simulink model "motor_foc"  (R2023b)
settings: Solver=FixedStepDiscrete  StartTime=0.0  StopTime=4  FixedStep=Ts  RelTol=1e-3  EnableMultiTasking=on
PreLoadFcn:
  | addpath(pwd);
InitFcn:
  | mc_init;
values from neighbouring files (symbols this model uses):
  ADC_Trigger = ADC_Trigger_Top    (= 1)    [mc_init.m]
  B = 0.000    (= 0)    [mc_init.m]
  Cdc = 470e-9    (= 4.7e-07)    [mc_init.m]
  Cphase = 2.2e-9    (= 2.2e-09)    [mc_init.m]
  enc_cpr = 4095    [mc_init.m]
  J = 0.020    (= 0.02)    [mc_init.m]
  Ld = 0.043e-3    (= 4.3e-05)    [mc_init.m]
  Lq = 0.060e-3    (= 6e-05)    [mc_init.m]
  n_polePairs = 5    [mc_init.m]
  PWM_Half_Cnt = PWM_Cnt/2    (= 3000)    [mc_init.m]
  R1 = 400e3    (= 400000)    [mc_init.m]
  R2 = 12e3    (= 12000)    [mc_init.m]
  Rdc = 2000    [mc_init.m]
  Rphase = 120    [mc_init.m]
  Rs = 0.015    [mc_init.m]
  Rshut = 0.001    [mc_init.m]
  TIMER_PWM_MODE = PWM_MODE1    (= 1)    [mc_init.m]
  Ts = 5e-7    (= 5e-07)    [mc_init.m]
  Ts_ctrl = 100e-6    (= 0.0001)    [mc_init.m]
  Udc = 96    [mc_init.m]
  Vbus_C = 3000e-6    (= 0.003)    [mc_init.m]
undefined symbols (not defined in the file or in its folder): Phase_Vol_R1
libraries: spsSeriesRLCBranchLib x9, spsIGBTDiodeLib x6, spsParallelRLCBranchLib x4, spsVoltageMeasurementLib x4, simulink x3, spsControlledVoltageSourceLib x1, spsPermanentMagnetSynchronousMachineLib x1, sps_lib x1
settings Model: Creator=kevin  LastModifiedBy=huhui
settings SolverCC: AlgebraicLoopSolver=TrustRegion  AutoInsertRateTranBlk=on
settings DebuggingCC: UnconnectedInputMsg=warning  UnconnectedOutputMsg=warning  UnconnectedLineMsg=warning
settings ModelReferenceCC: EnableRefExpFcnMdlSchedulingChecks=on
settings RTWCC: DLArmComputeVersion=19.05

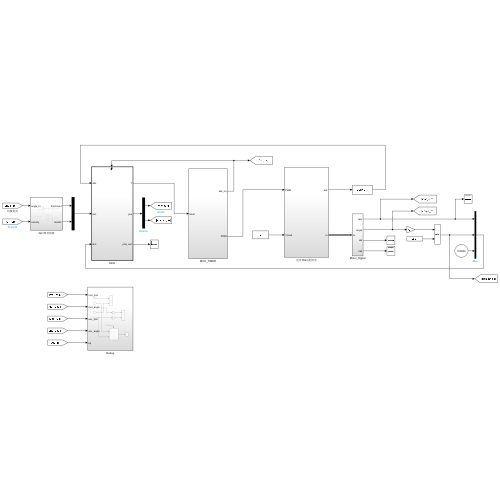
[thumbnail: Simulink's stored preview of the top-level diagram]
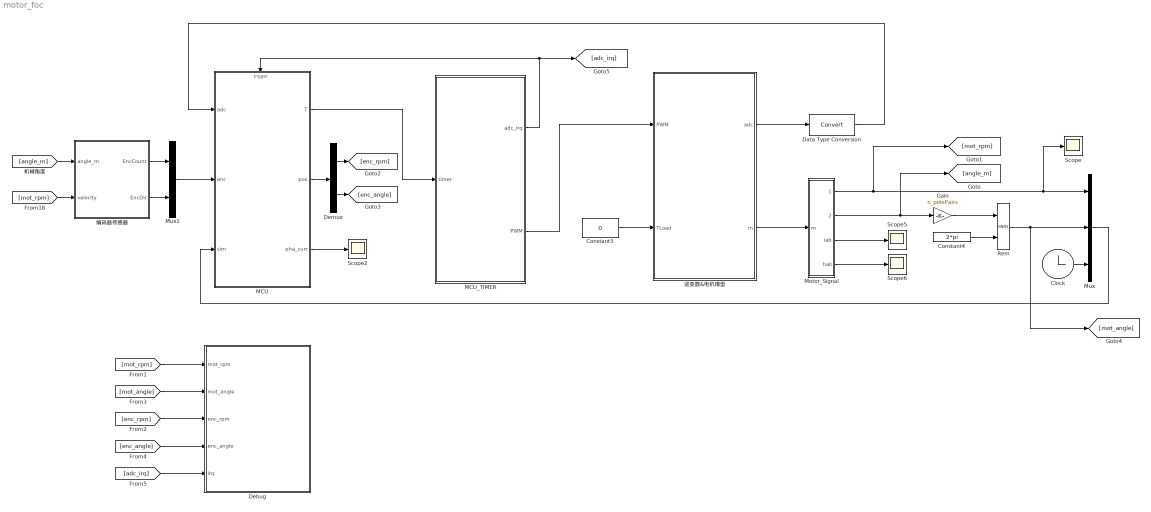
== system motor_foc ==
  Clock : Clock
  Constant3 : Constant  Value=0
  Constant4 : Constant  Value=2*pi
  Data Type Conversion : DataTypeConversion  SaturateOnIntegerOverflow=off  RndMeth=Floor
  Debug : Subsystem
  Demux : Demux  Outputs=2
  Gain : Gain  Gain=n_polePairs
  MCU : Subsystem  TreatAsAtomicUnit=on
  MCU_TIMER : Subsystem
  Motor_Signal : Subsystem
  Mux : Mux  Inputs=3
  Mux1 : Mux  Inputs=2
  Rem : Math  Operator=rem
  Scope{,2,5..6} (4 alike) : Scope
  编码器传感器 : Subsystem
  逆变器&电机模型 : Subsystem
  wires:
  MCU/1(T) -> MCU_TIMER/1(timer)
  MCU/2(pos) -> Demux/1
  MCU/3(pha_curr) -> Scope2/1
  MCU_TIMER/2(PWM) -> 逆变器&电机模型/1(PWM)
  MCU_TIMER/1(adc_irq) -> [adc_irq], MCU/Trigger
  逆变器&电机模型/2(m) -> Motor_Signal/1(m)
  Constant3/1 -> 逆变器&电机模型/2(TLoad)
  逆变器&电机模型/1(adc) -> Data Type Conversion/1
  Motor_Signal/1(rpm) -> Mux/1, Scope/1, [mot_rpm]
  Motor_Signal/3(iab) -> Scope5/1
  Motor_Signal/4(hall) -> Scope6/1
  Gain/1 -> Rem/1
  Constant4/1 -> Rem/2
  Motor_Signal/2(angle) -> [angle_m], Gain/1
  Rem/1 -> [mot_angle], Mux/2
  Clock/1 -> Mux/3
  Mux/1 -> MCU/3(sim)
  Data Type Conversion/1 -> MCU/1(adc)
  编码器传感器/2(EncDir) -> Mux1/2
  编码器传感器/1(EncCount) -> Mux1/1
  [mot_rpm] -> 编码器传感器/2(velocity)
  [angle_m] -> 编码器传感器/1(angle_m)
  Mux1/1 -> MCU/2(enc)
  Demux/2 -> [enc_angle]
  Demux/1 -> [enc_rpm]
  [adc_irq] -> Debug/5(irq)
  [mot_rpm] -> Debug/1(mot_rpm)
  [mot_angle] -> Debug/2(mot_angle)
  [enc_rpm] -> Debug/3(enc_rpm)
  [enc_angle] -> Debug/4(enc_angle)

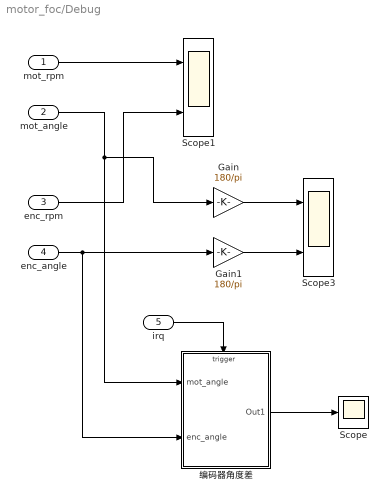
== system motor_foc/Debug ==
  mot_rpm : Inport
  mot_angle : Inport  Port=2
  enc_rpm : Inport  Port=3
  enc_angle : Inport  Port=4
  irq : Inport  Port=5
  Gain : Gain  Gain=180/pi
  Gain1 : Gain  Gain=180/pi
  Scope : Scope
  Scope1 : Scope  NumInputPorts=2
  Scope3 : Scope  NumInputPorts=2
  编码器角度差 : Subsystem
  wires:
  mot_angle/1 -> 编码器角度差/1(mot_angle), Gain/1
  编码器角度差/1(Out1) -> Scope/1
  enc_angle/1 -> 编码器角度差/2(enc_angle), Gain1/1
  irq/1 -> 编码器角度差/Trigger
  mot_rpm/1 -> Scope1/1
  enc_rpm/1 -> Scope1/2
  Gain/1 -> Scope3/1
  Gain1/1 -> Scope3/2

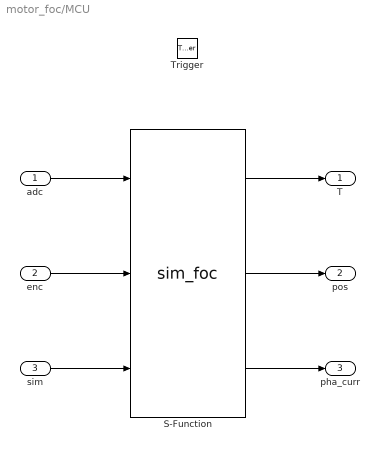
== system motor_foc/MCU ==
  adc : Inport
  enc : Inport  Port=2
  sim : Inport  Port=3
  Trigger : TriggerPort  VariantControl=(inherit)  PortDimensions=1
  S-Function : S-Function  FunctionName=sim_foc  SFunctionDeploymentMode=off  EnableBusSupport=off
  T : Outport
  pos : Outport  Port=2
  pha_curr : Outport  Port=3
  wires:
  adc/1 -> S-Function/1
  S-Function/1 -> T/1
  S-Function/2 -> pos/1
  S-Function/3 -> pha_curr/1
  sim/1 -> S-Function/3
  enc/1 -> S-Function/2

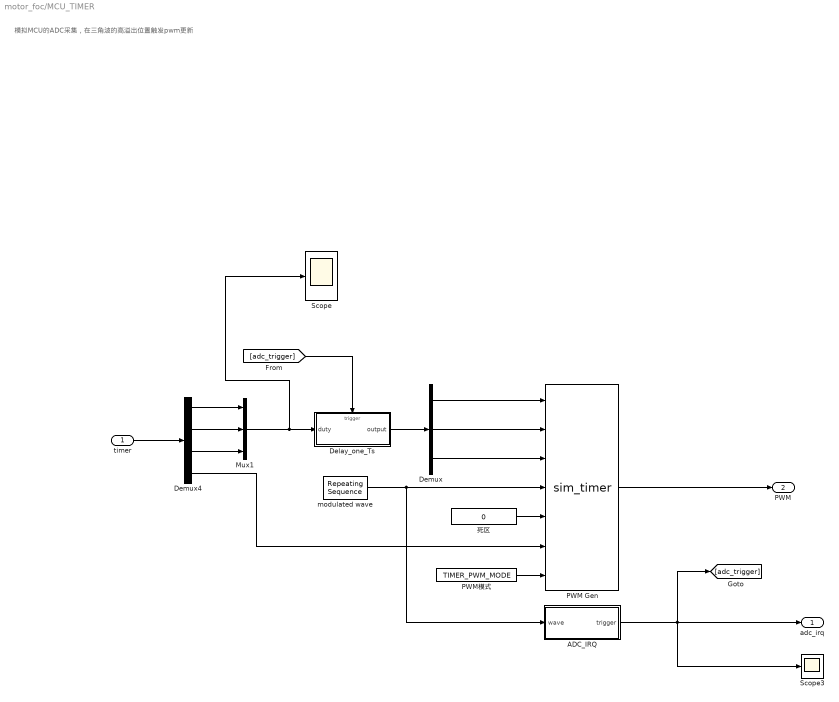
== system motor_foc/MCU_TIMER ==
  note: 模拟MCU的ADC采集，在三角波的高溢出位置触发pwm更新
  timer : Inport
  ADC_IRQ : Subsystem
  Delay_one_Ts : Subsystem  TreatAsAtomicUnit=on
  Demux : Demux  Outputs=3
  Demux4 : Demux
  Mux1 : Mux  Inputs=3
  PWM Gen : S-Function  FunctionName=sim_timer  SFunctionDeploymentMode=off  EnableBusSupport=off
  PWM模式 : Constant  Value=TIMER_PWM_MODE
  Scope : Scope
  Scope3 : Scope
  modulated wave : simulink/Sources/Repeating Sequence  rep_seq_t=[0 Ts_ctrl/2 Ts_ctrl]  rep_seq_y=[0 PWM_Half_Cnt 0]
  死区 : Constant  Value=0
  adc_irq : Outport
  PWM : Outport  Port=2
  wires:
  Demux/2 -> PWM Gen/2
  Demux/3 -> PWM Gen/3
  Demux/1 -> PWM Gen/1
  Delay_one_Ts/1(output) -> Demux/1
  [adc_trigger] -> Delay_one_Ts/Trigger
  死区/1 -> PWM Gen/5
  PWM Gen/1 -> PWM/1
  modulated wave/1 -> ADC_IRQ/1(wave), PWM Gen/4
  Mux1/1 -> Scope/1, Delay_one_Ts/1(duty)
  Demux4/3 -> Mux1/3
  Demux4/2 -> Mux1/2
  Demux4/1 -> Mux1/1
  timer/1 -> Demux4/1
  Demux4/4 -> PWM Gen/6
  ADC_IRQ/1(trigger) -> Scope3/1, [adc_trigger], adc_irq/1
  PWM模式/1 -> PWM Gen/7

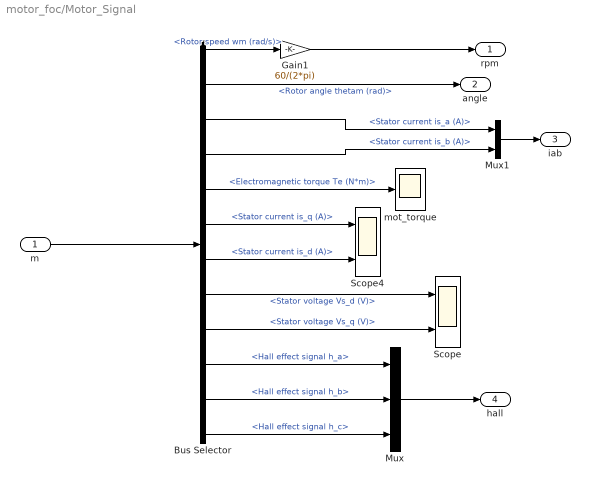
== system motor_foc/Motor_Signal ==
  m : Inport
  " mot_torque" : Scope
  Bus Selector : BusSelector  OutputSignals=Rotor speed wm (rad/s),Rotor angle thetam (rad),Stator current is_a (A),Stator current is_b (A),Electromagnetic torque Te (N*m),Stator current is_q (A),Stator current is_d (A),Stator voltage Vs_d (V),Stator voltage Vs_q (V),Hall effect signal h_a,Hall effect signal h_b,Hall effect signal h_c
  Gain1 : Gain  Gain=60/(2*pi)
  Mux : Mux  Inputs=3
  Mux1 : Mux  Inputs=2
  Scope : Scope  NumInputPorts=2
  Scope4 : Scope  NumInputPorts=2
  rpm : Outport
  angle : Outport  Port=2
  iab : Outport  Port=3
  hall : Outport  Port=4
  wires:
  Bus Selector/8 -> Scope/1  "<Stator voltage Vs_d (V)>"
  Bus Selector/2 -> angle/1  "<Rotor angle thetam (rad)>"
  Bus Selector/7 -> Scope4/2  "<Stator current is_d (A)>"
  Bus Selector/5 -> " mot_torque"/1  "<Electromagnetic torque Te (N*m)>"
  Bus Selector/6 -> Scope4/1  "<Stator current is_q (A)>"
  Bus Selector/1 -> Gain1/1  "<Rotor speed wm (rad/s)>"
  Bus Selector/9 -> Scope/2  "<Stator voltage Vs_q (V)>"
  m/1 -> Bus Selector/1
  Gain1/1 -> rpm/1
  Bus Selector/4 -> Mux1/2  "<Stator current is_b (A)>"
  Bus Selector/10 -> Mux/1  "<Hall effect signal h_a>"
  Bus Selector/11 -> Mux/2  "<Hall effect signal h_b>"
  Bus Selector/12 -> Mux/3  "<Hall effect signal h_c>"
  Mux/1 -> hall/1
  Bus Selector/3 -> Mux1/1  "<Stator current is_a (A)>"
  Mux1/1 -> iab/1

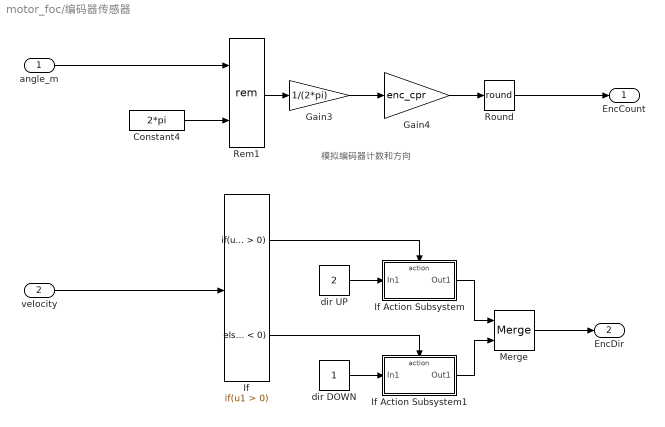
== system motor_foc/编码器传感器 ==
  note: 模拟编码器计数和方向
  angle_m : Inport
  velocity : Inport  Port=2
  Constant4 : Constant  Value=2*pi
  Gain3 : Gain  Gain=1/(2*pi)
  Gain4 : Gain  Gain=enc_cpr
  If : If  ElseIfExpressions=u1 < 0  ShowElse=off
  If Action Subsystem : Subsystem  TreatAsAtomicUnit=on
  If Action Subsystem1 : Subsystem  TreatAsAtomicUnit=on
  Merge : Merge
  Rem1 : Math  Operator=rem
  Round : Rounding  Operator=round
  dir DOWN : Constant
  dir UP : Constant  Value=2
  EncCount : Outport
  EncDir : Outport  Port=2
  wires:
  angle_m/1 -> Rem1/1
  Gain4/1 -> Round/1
  If Action Subsystem/1(Out1) -> Merge/1
  Gain3/1 -> Gain4/1
  If Action Subsystem1/1(Out1) -> Merge/2
  dir DOWN/1 -> If Action Subsystem1/1(In1)
  If/1 -> If Action Subsystem/Action
  If/2 -> If Action Subsystem1/Action
  Constant4/1 -> Rem1/2
  dir UP/1 -> If Action Subsystem/1(In1)
  Rem1/1 -> Gain3/1
  Round/1 -> EncCount/1
  velocity/1 -> If/1
  Merge/1 -> EncDir/1

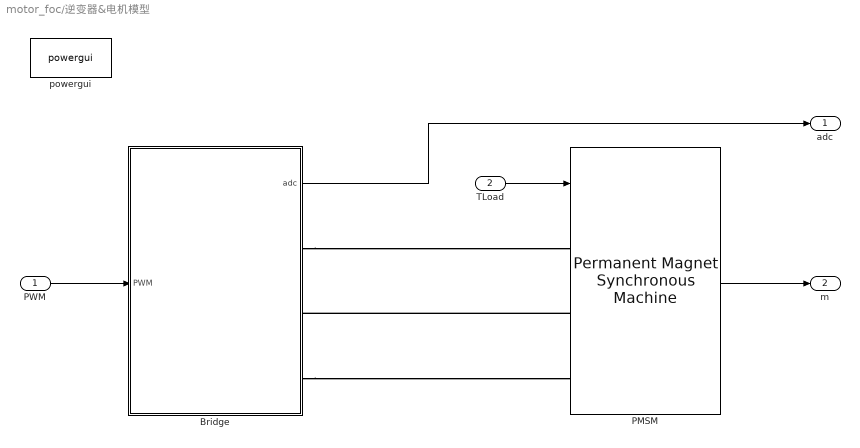
== system motor_foc/逆变器&电机模型 ==
  PWM : Inport
  TLoad : Inport  Port=2
  Bridge : Subsystem
  PMSM : spsPermanentMagnetSynchronousMachineLib/Permanent Magnet Synchronous Machine  NbPhases=3  FluxDistribution=Sinusoidal  RotorType=Salient-pole  MechanicalLoad=Torque Tm  PresetModel=No  ShowDetailedParameters=on  MeasurementBus=off  Resistance=Rs  Inductance=8.5e-3  dqInductances=[Ld Lq]  La=Ls  MachineConstant=Flux linkage established by magnets (V.s)  Flux=PM  VoltageCst=16.3242  TorqueCst=0.135  Flat=120  Mechanical=[J B n_polePairs 0]  PolePairs=n_polePairs  InitialConditions=[0, 0, 0,0]  InitialConditions5ph=[0 0 0 0 0 0]  RefAngle=Aligned with phase A axis (original Park)  IterativeDiscreteModel=Trapezoidal non iterative  TsBlock=-1  TsPowergui=0
  powergui : sps_lib/powergui  Priority=1  SimulationMode=Discrete  SampleTime=Ts  frequency=60  Iterations=50  frequencyindice=0  Pbase=100e6  ErrMax=1e-4  UnitsV=kV  UnitsW=MW  buscounter=0  FunctionMessages=off  echomessages=off  EnableUseOfTLC=off  CurrentSourceSwitches=off  DisableSnubberDevices=off  DisableRonSwitches=off  DisableVfSwitches=off  DisplayEquations=off  AutomaticDiscreteSolvers=on  SolverType=Tustin/Backward Euler (TBE)  Interpol=off  ExternalGateDelay=off  methode=off  Ts=100  x0status=blocks  SPID=on  SwTol=0  HookPort=off  NonlinearTolerance=1e-6  nMaxIteration=1000  ContinueOnMaxIteration=off  RestoreLinks=warning  ResistiveCurrentMeasurement=off  Frange=[0:2:500]  Ylog=off  Xlog=on  ShowGrid=off  save=off  variable=ZData  structure=0  ZoomFFT=off  StartTime=0.0  cycles=1  DisplayStyle=1  fundamental=60  FreqAxis=off  MaxFrequency=1000  frequencyindicesteady=1  RmsSteady=1  display=off
  adc : Outport
  m : Outport  Port=2
  wires:
  PWM/1 -> Bridge/1(PWM)
  TLoad/1 -> PMSM/1
  PMSM/1 -> m/1
  Bridge/1(adc) -> adc/1
  connections:
  PMSM/LConn2 -- Bridge/RConn2
  Bridge/RConn1 -- PMSM/LConn1
  Bridge/RConn3 -- PMSM/LConn3

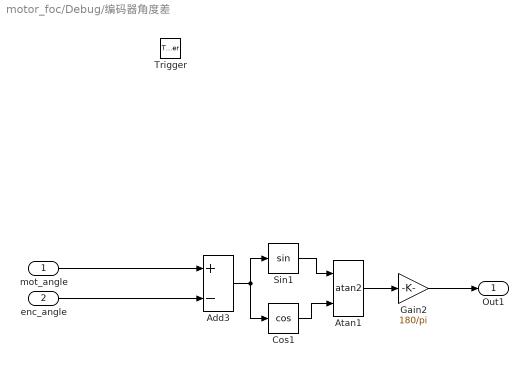
== system motor_foc/Debug/编码器角度差 ==
  mot_angle : Inport
  enc_angle : Inport  Port=2
  Trigger : TriggerPort  VariantControl=Variant  PortDimensions=1
  Add3 : Sum  Inputs=+-
  Atan1 : Trigonometry  Operator=atan2
  Cos1 : Trigonometry  Operator=cos
  Gain2 : Gain  Gain=180/pi
  Sin1 : Trigonometry
  Out1 : Outport
  wires:
  mot_angle/1 -> Add3/1
  Sin1/1 -> Atan1/1
  Gain2/1 -> Out1/1
  Atan1/1 -> Gain2/1
  Cos1/1 -> Atan1/2
  enc_angle/1 -> Add3/2
  Add3/1 -> Sin1/1, Cos1/1

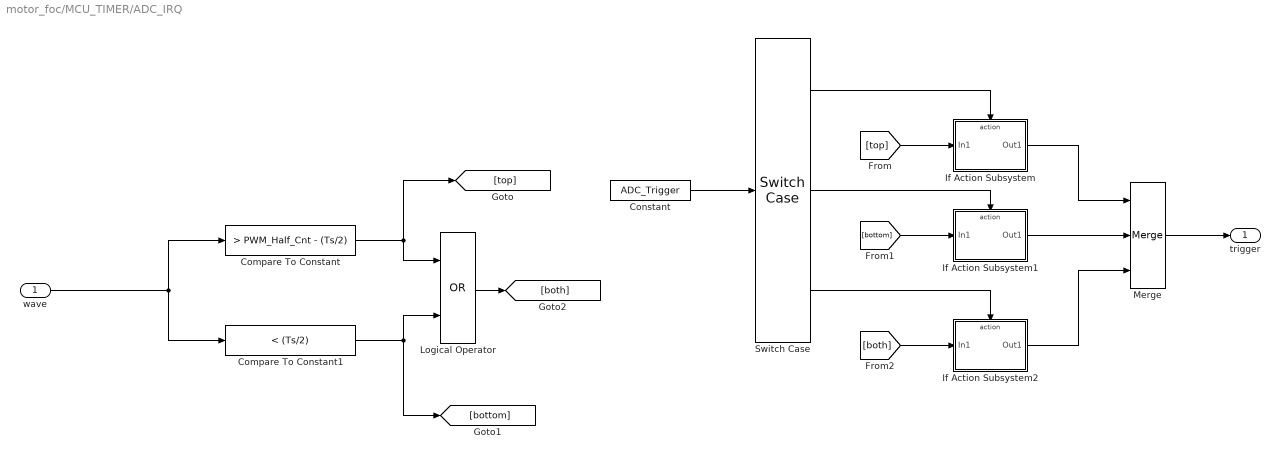
== system motor_foc/MCU_TIMER/ADC_IRQ ==
  wave : Inport
  Compare To Constant : simulink/Logic and Bit Operations/Compare To Constant  relop=>  const=PWM_Half_Cnt - (Ts/2)  OutDataTypeStr=boolean
  Compare To Constant1 : simulink/Logic and Bit Operations/Compare To Constant  relop=<  const=(Ts/2)  OutDataTypeStr=boolean
  Constant : Constant  Value=ADC_Trigger
  If Action Subsystem : Subsystem  TreatAsAtomicUnit=on
  If Action Subsystem1 : Subsystem  TreatAsAtomicUnit=on
  If Action Subsystem2 : Subsystem  TreatAsAtomicUnit=on
  Logical Operator : Logic  Operator=OR  AllPortsSameDT=off  OutDataTypeStr=boolean
  Merge : Merge  Inputs=3
  Switch Case : SwitchCase  CaseConditions={1,2,3}  ShowDefaultCase=off
  trigger : Outport
  wires:
  wave/1 -> Compare To Constant1/1, Compare To Constant/1
  Compare To Constant/1 -> Logical Operator/1, [top]
  Compare To Constant1/1 -> [bottom], Logical Operator/2
  Switch Case/1 -> If Action Subsystem/Action
  Logical Operator/1 -> [both]
  Constant/1 -> Switch Case/1
  [top] -> If Action Subsystem/1(In1)
  Switch Case/2 -> If Action Subsystem1/Action
  [bottom] -> If Action Subsystem1/1(In1)
  Switch Case/3 -> If Action Subsystem2/Action
  [both] -> If Action Subsystem2/1(In1)
  If Action Subsystem/1(Out1) -> Merge/1
  If Action Subsystem1/1(Out1) -> Merge/2
  If Action Subsystem2/1(Out1) -> Merge/3
  Merge/1 -> trigger/1

== system motor_foc/MCU_TIMER/Delay_one_Ts ==
  duty : Inport
  Trigger : TriggerPort  VariantControl=Variant
  output : Outport
  wires:
  duty/1 -> output/1

== system motor_foc/编码器传感器/If Action Subsystem ==
  In1 : Inport
  Action Port : ActionPort  ActionPortLabel=if(u1 > 0)
  Out1 : Outport
  wires:
  In1/1 -> Out1/1

== system motor_foc/编码器传感器/If Action Subsystem1 ==
  In1 : Inport
  Action Port : ActionPort  ActionPortLabel=elseif(u1 < 0)
  Out1 : Outport
  wires:
  In1/1 -> Out1/1

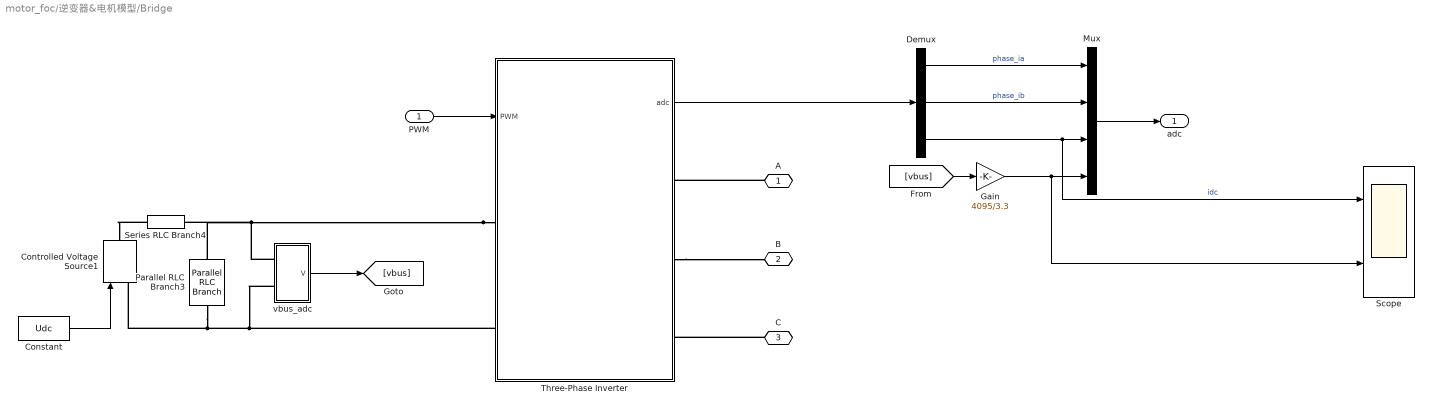
== system motor_foc/逆变器&电机模型/Bridge ==
  PWM : Inport
  Constant : Constant  Value=Udc
  Controlled Voltage Source1 : spsControlledVoltageSourceLib/Controlled Voltage Source  Initialize=on  Source_Type=DC  Amplitude=0  Phase=0  Frequency=0  Measurements=None
  Demux : Demux  Outputs=3
  Gain : Gain  Gain=4095/3.3  OutDataTypeStr=int32
  Mux : Mux
  Parallel RLC Branch3 : spsParallelRLCBranchLib/Parallel RLC Branch  LConnTagsString=a  RConnTagsString=__new0  BranchType=C  Resistance=Phase_Vol_R1  Inductance=1e-3  SetiL0=off  InitialCurrent=0  Capacitance=Vbus_C  Setx0=off  InitialVoltage=0  Measurements=None
  Scope : Scope  NumInputPorts=2
  Series RLC Branch4 : spsSeriesRLCBranchLib/Series RLC Branch  LConnTagsString=__new0  RConnTagsString=__new0  BranchType=R  Resistance=1e-5  Inductance=1e-3  SetiL0=off  InitialCurrent=0  Capacitance=1e-6  Setx0=off  InitialVoltage=0  Measurements=None
  Three-Phase Inverter : Subsystem
  vbus_adc : Subsystem
  A : PMIOPort  Side=Right
  B : PMIOPort  Port=2  Side=Right
  C : PMIOPort  Port=3  Side=Right
  adc : Outport
  wires:
  PWM/1 -> Three-Phase Inverter/1(PWM)
  Constant/1 -> Controlled Voltage Source1/1
  Three-Phase Inverter/1(adc) -> Demux/1
  Demux/2 -> Mux/2  "phase_ib"
  Demux/1 -> Mux/1  "phase_ia"
  Demux/3 -> Scope/1, Mux/3  "idc"
  Mux/1 -> adc/1
  vbus_adc/1(V) -> [vbus]
  [vbus] -> Gain/1
  Gain/1 -> Scope/2, Mux/4
  connections:
  A/RConn1 -- Three-Phase Inverter/RConn1
  Three-Phase Inverter/LConn2 -- vbus_adc/LConn2 -- Controlled Voltage Source1/LConn1 -- Parallel RLC Branch3/RConn1
  Three-Phase Inverter/RConn2 -- B/RConn1
  Three-Phase Inverter/LConn1 -- vbus_adc/LConn1 -- Series RLC Branch4/RConn1 -- Parallel RLC Branch3/LConn1
  C/RConn1 -- Three-Phase Inverter/RConn3
  Series RLC Branch4/LConn1 -- Controlled Voltage Source1/RConn1

== system motor_foc/MCU_TIMER/ADC_IRQ/If Action Subsystem ==
  In1 : Inport
  Action Port : ActionPort  ActionPortLabel=case [ 1 ]:
  Out1 : Outport
  wires:
  In1/1 -> Out1/1

== system motor_foc/MCU_TIMER/ADC_IRQ/If Action Subsystem1 ==
  In1 : Inport
  Action Port : ActionPort  ActionPortLabel=case [ 2 ]:
  Out1 : Outport
  wires:
  In1/1 -> Out1/1

== system motor_foc/MCU_TIMER/ADC_IRQ/If Action Subsystem2 ==
  In1 : Inport
  Action Port : ActionPort  ActionPortLabel=case [ 3 ]:
  Out1 : Outport
  wires:
  In1/1 -> Out1/1

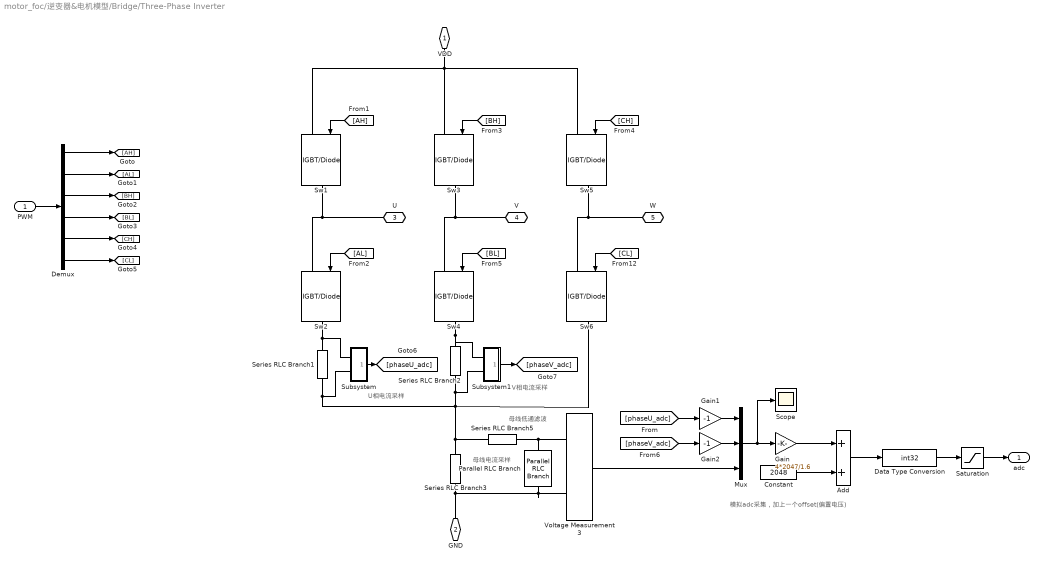
== system motor_foc/逆变器&电机模型/Bridge/Three-Phase Inverter ==
  note: 模拟adc采集，加上一个offset(偏置电压)
  note: V相电流采样
  note: U相电流采样
  note: 母线电流采样
  note: 母线低通滤波
  PWM : Inport
  Add : Sum
  Constant : Constant  Value=2048
  Data Type Conversion : DataTypeConversion  OutDataTypeStr=int32  SaturateOnIntegerOverflow=off  RndMeth=Floor
  Demux : Demux  Outputs=6
  Gain : Gain  Gain=4*2047/1.6
  Gain1 : Gain  Gain=-1
  Gain2 : Gain  Gain=-1
  Mux : Mux  Inputs=3
  Parallel RLC Branch : spsParallelRLCBranchLib/Parallel RLC Branch  LConnTagsString=a  RConnTagsString=__new0  BranchType=C  Resistance=Phase_Vol_R1  Inductance=1e-3  SetiL0=off  InitialCurrent=0  Capacitance=Cdc  Setx0=off  InitialVoltage=0  Measurements=None
  Saturation : Saturate  UpperLimit=4095  LowerLimit=0
  Scope : Scope
  Series RLC Branch1 : spsSeriesRLCBranchLib/Series RLC Branch  LConnTagsString=__new0  RConnTagsString=__new0  BranchType=R  Resistance=Rshut  Inductance=1e-3  SetiL0=off  InitialCurrent=0  Capacitance=1e-6  Setx0=off  InitialVoltage=0  Measurements=None
  Series RLC Branch2 : spsSeriesRLCBranchLib/Series RLC Branch  LConnTagsString=__new0  RConnTagsString=__new0  BranchType=R  Resistance=Rshut  Inductance=1e-3  SetiL0=off  InitialCurrent=0  Capacitance=1e-6  Setx0=off  InitialVoltage=0  Measurements=None
  Series RLC Branch3 : spsSeriesRLCBranchLib/Series RLC Branch  LConnTagsString=__new0  RConnTagsString=__new0  BranchType=R  Resistance=Rshut  Inductance=1e-3  SetiL0=off  InitialCurrent=0  Capacitance=1e-6  Setx0=off  InitialVoltage=0  Measurements=None
  Series RLC Branch5 : spsSeriesRLCBranchLib/Series RLC Branch  LConnTagsString=__new0  RConnTagsString=__new0  BranchType=R  Resistance=Rdc  Inductance=1e-3  SetiL0=off  InitialCurrent=0  Capacitance=1e-6  Setx0=off  InitialVoltage=0  Measurements=None
  Subsystem : Subsystem
  Subsystem1 : Subsystem
  Sw{1..6} (6 alike) : spsIGBTDiodeLib/IGBT//Diode  Ron=1e-3  Rs=1e6  Cs=inf  Measurements=off
  Voltage Measurement3 : spsVoltageMeasurementLib/Voltage Measurement  PhasorSimulation=off  OutputType=Complex  PSBequivalent=0
  VDD : PMIOPort  Side=Left
  GND : PMIOPort  Port=2  Side=Left
  U : PMIOPort  Port=3  Side=Right
  V : PMIOPort  Port=4  Side=Right
  W : PMIOPort  Port=5  Side=Right
  adc : Outport
  wires:
  Gain2/1 -> Mux/2
  Gain1/1 -> Mux/1
  Saturation/1 -> adc/1
  Data Type Conversion/1 -> Saturation/1
  Mux/1 -> Gain/1, Scope/1
  Voltage Measurement3/1 -> Mux/3
  [phaseV_adc] -> Gain2/1
  [phaseU_adc] -> Gain1/1
  Subsystem1/1(V) -> [phaseV_adc]
  [CL] -> Sw6/1
  [BL] -> Sw4/1
  [CH] -> Sw5/1
  [BH] -> Sw3/1
  [AL] -> Sw2/1
  [AH] -> Sw1/1
  Demux/5 -> [CH]
  Demux/6 -> [CL]
  Demux/3 -> [BH]
  Demux/4 -> [BL]
  Demux/2 -> [AL]
  Demux/1 -> [AH]
  PWM/1 -> Demux/1
  Constant/1 -> Add/2
  Gain/1 -> Add/1
  Add/1 -> Data Type Conversion/1
  Subsystem/1(V) -> [phaseU_adc]
  connections:
  Parallel RLC Branch/LConn1 -- Series RLC Branch5/RConn1 -- Voltage Measurement3/LConn1
  Series RLC Branch3/RConn1 -- Parallel RLC Branch/RConn1 -- Voltage Measurement3/LConn2 -- GND/RConn1
  Sw4/RConn1 -- Subsystem1/LConn1 -- Series RLC Branch2/LConn1
  Sw2/RConn1 -- Subsystem/LConn1 -- Series RLC Branch1/LConn1
  Sw5/LConn1 -- Sw3/LConn1 -- VDD/RConn1 -- Sw1/LConn1
  Series RLC Branch2/RConn1 -- Sw6/RConn1 -- Subsystem/LConn2 -- Series RLC Branch1/RConn1 -- Series RLC Branch5/LConn1 -- Series RLC Branch3/LConn1 -- Subsystem1/LConn2
  W/RConn1 -- Sw6/LConn1 -- Sw5/RConn1
  V/RConn1 -- Sw4/LConn1 -- Sw3/RConn1
  Sw2/LConn1 -- U/RConn1 -- Sw1/RConn1

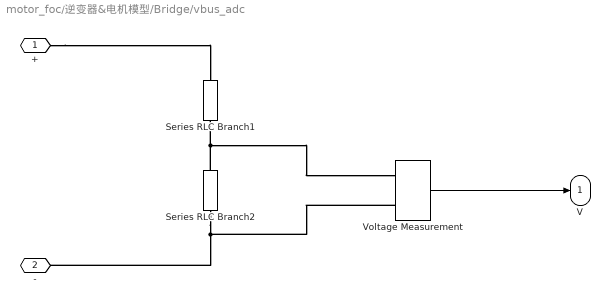
== system motor_foc/逆变器&电机模型/Bridge/vbus_adc ==
  Series RLC Branch1 : spsSeriesRLCBranchLib/Series RLC Branch  LConnTagsString=__new0  RConnTagsString=__new0  BranchType=R  Resistance=R1  Inductance=1e-3  SetiL0=off  InitialCurrent=0  Capacitance=1e-6  Setx0=off  InitialVoltage=0  Measurements=None
  Series RLC Branch2 : spsSeriesRLCBranchLib/Series RLC Branch  LConnTagsString=__new0  RConnTagsString=__new0  BranchType=R  Resistance=R2  Inductance=1e-3  SetiL0=off  InitialCurrent=0  Capacitance=1e-6  Setx0=off  InitialVoltage=0  Measurements=None
  Voltage Measurement : spsVoltageMeasurementLib/Voltage Measurement  PhasorSimulation=off  OutputType=Complex  PSBequivalent=0
  + : PMIOPort  Side=Left
  - : PMIOPort  Port=2  Side=Left
  V : Outport
  wires:
  Voltage Measurement/1 -> V/1
  connections:
  Series RLC Branch2/RConn1 -- -/RConn1 -- Voltage Measurement/LConn2
  Series RLC Branch2/LConn1 -- Voltage Measurement/LConn1 -- Series RLC Branch1/RConn1
  +/RConn1 -- Series RLC Branch1/LConn1

== system motor_foc/逆变器&电机模型/Bridge/Three-Phase Inverter/Subsystem ==
  Parallel RLC Branch1 : spsParallelRLCBranchLib/Parallel RLC Branch  LConnTagsString=a  RConnTagsString=__new0  BranchType=C  Resistance=Phase_Vol_R1  Inductance=1e-3  SetiL0=off  InitialCurrent=0  Capacitance=Cphase  Setx0=off  InitialVoltage=0  Measurements=None
  Series RLC Branch6 : spsSeriesRLCBranchLib/Series RLC Branch  LConnTagsString=__new0  RConnTagsString=__new0  BranchType=R  Resistance=Rphase  Inductance=1e-3  SetiL0=off  InitialCurrent=0  Capacitance=1e-6  Setx0=off  InitialVoltage=0  Measurements=None
  Voltage Measurement1 : spsVoltageMeasurementLib/Voltage Measurement  PhasorSimulation=off  OutputType=Complex  PSBequivalent=0
  + : PMIOPort  Side=Left
  - : PMIOPort  Port=2  Side=Left
  V : Outport
  wires:
  Voltage Measurement1/1 -> V/1
  connections:
  Series RLC Branch6/LConn1 -- +/RConn1
  Series RLC Branch6/RConn1 -- Voltage Measurement1/LConn1 -- Parallel RLC Branch1/LConn1
  Parallel RLC Branch1/RConn1 -- Voltage Measurement1/LConn2 -- -/RConn1

== system motor_foc/逆变器&电机模型/Bridge/Three-Phase Inverter/Subsystem1 ==
  Parallel RLC Branch1 : spsParallelRLCBranchLib/Parallel RLC Branch  LConnTagsString=a  RConnTagsString=__new0  BranchType=C  Resistance=Phase_Vol_R1  Inductance=1e-3  SetiL0=off  InitialCurrent=0  Capacitance=Cphase  Setx0=off  InitialVoltage=0  Measurements=None
  Series RLC Branch6 : spsSeriesRLCBranchLib/Series RLC Branch  LConnTagsString=__new0  RConnTagsString=__new0  BranchType=R  Resistance=Rphase  Inductance=1e-3  SetiL0=off  InitialCurrent=0  Capacitance=1e-6  Setx0=off  InitialVoltage=0  Measurements=None
  Voltage Measurement1 : spsVoltageMeasurementLib/Voltage Measurement  PhasorSimulation=off  OutputType=Complex  PSBequivalent=0
  + : PMIOPort  Side=Left
  - : PMIOPort  Port=2  Side=Left
  V : Outport
  wires:
  Voltage Measurement1/1 -> V/1
  connections:
  -/RConn1 -- Voltage Measurement1/LConn2 -- Parallel RLC Branch1/RConn1
  Parallel RLC Branch1/LConn1 -- Voltage Measurement1/LConn1 -- Series RLC Branch6/RConn1
  Series RLC Branch6/LConn1 -- +/RConn1
